simulink model "ackerman_purepursuit"  (R2023b)
settings: Solver=VariableStepAuto  StartTime=0.0  StopTime=9  RelTol=1e-3
model workspace (MAT data in the model file):
  distfw = 0.0267
  distrw = 0.0267
  robot_radius = 0.0639
  wheelrad = 0.004
libraries: mobileRoboticsLib x3, robotalgslib x1
settings Model: Creator=mihai  LastModifiedBy=mihai

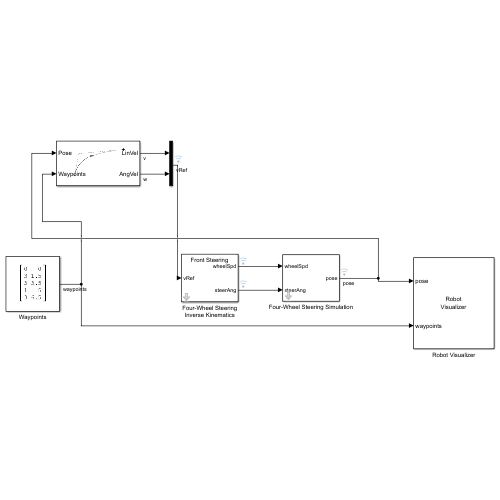
[thumbnail: Simulink's stored preview of the top-level diagram]
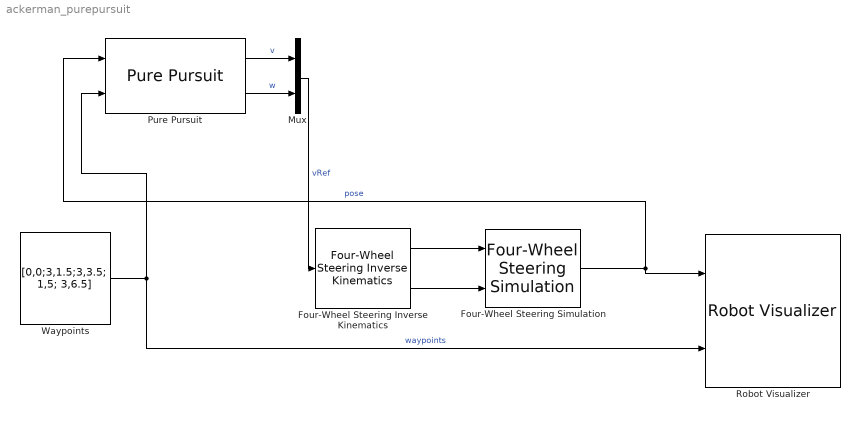
== system ackerman_purepursuit ==
  Four-Wheel Steering Inverse Kinematics : mobileRoboticsLib/Kinematic Models/Four-Wheel Steering/Four-Wheel Steering Inverse Kinematics  wheelRadius=wheelrad  frontWheelDist=distfw  rearWheelDist=distrw  ikMode=Front Steering
      settings: SourceProductName=Mobile Robotics Simulation Toolbox
  Four-Wheel Steering Simulation : mobileRoboticsLib/Kinematic Models/Four-Wheel Steering/Four-Wheel Steering Simulation  wheelRadius=wheelrad  frontWheelDist=distfw  rearWheelDist=distrw  initX=0  initY=0  initAngle=0  Ts=0.05
      settings: SourceProductName=Mobile Robotics Simulation Toolbox
  Mux : Mux  Inputs=2
  Pure Pursuit : robotalgslib/Pure Pursuit  DesiredLinearVelocity=1.2  MaxAngularVelocity=22.47  LookaheadDistance=0.3  TargetDirPort=off  SimulateUsing=Interpreted execution
  Robot Visualizer : mobileRoboticsLib/Environments/Robot Visualizer  Priority=99  robotRadius=robot_radius  showTrajectory=on  hasWaypoints=on  hasLidar=off  sensorOffset=[ 0 0 ]  scanAngles=0  hasObjDetector=off  objDetectorOffset=[ 0, 0 ]  objDetectorAngle=0  objDetectorFOV=0  objDetectorMaxRange=0  objectColors=0  objectMarkers=s
  Waypoints : Constant  Value=[0,0;3,1.5;3,3.5; 1,5; 3,6.5]
  wires:
  Four-Wheel Steering Inverse Kinematics/1 -> Four-Wheel Steering Simulation/1
  Four-Wheel Steering Inverse Kinematics/2 -> Four-Wheel Steering Simulation/2
  Four-Wheel Steering Simulation/1 -> Pure Pursuit/1, Robot Visualizer/1  "pose"
  Waypoints/1 -> Pure Pursuit/2, Robot Visualizer/2  "waypoints"
  Pure Pursuit/1 -> Mux/1  "v"
  Pure Pursuit/2 -> Mux/2  "w"
  Mux/1 -> Four-Wheel Steering Inverse Kinematics/1  "vRef"
